simulink model "ex4sima"  (R2018a)
settings: Solver=ode45  StartTime=0.0  StopTime=10  RelTol=1e-3  EnableMultiTasking=on
values from neighbouring files (symbols this model uses):
  A = double(subs(A_sym, symbs, vals))    [load_params.m]
  B = double(subs(B_sym, symbs, vals))    [load_params.m]
  C = double(subs(C_sym, symbs, vals))    [load_params.m]    (also in load_pwm_avg_pred_controller.m = sysd.c; load_pwm_pred_controller.m = sysd.c)
undefined symbols (not defined in the file or in its folder): Ts
settings Model: Creator=BPeixoto  LastModifiedBy=brunolnetto
settings DataIOCC: LimitDataPoints=on  SaveFormat=Array
settings OptimizationCC: LifeSpan=inf
settings DebuggingCC: SFUnexpectedBacktrackingDiag=warning  SFNoUnconditionalDefaultTransitionDiag=warning  SFExecutionAtInitializationDiag=none
settings HardwareCC: ProdBitPerPointer=32  ProdBitPerSizeT=32  ProdBitPerPtrDiffT=32  ProdLargestAtomicFloat=None  ProdIntDivRoundTo=Undefined  ProdEndianess=Unspecified  ProdWordSize=32  ProdHWDeviceType=32-bit Generic
settings ModelReferenceCC: PropagateSignalLabelsOutOfModel=off
settings CodeAppCC: StateflowObjectComments=on
settings GRTTargetCC: TargetLangStandard=C89/C90 (ANSI)  GeneratePreprocessorConditionals=Disable all
settings ConfigComp: CovMetricSettings=dw  CovHtmlReporting=on  CovSaveCumulativeToWorkspaceVar=on  CovSaveSingleToWorkspaceVar=on  CovExternalEMLEnable=off

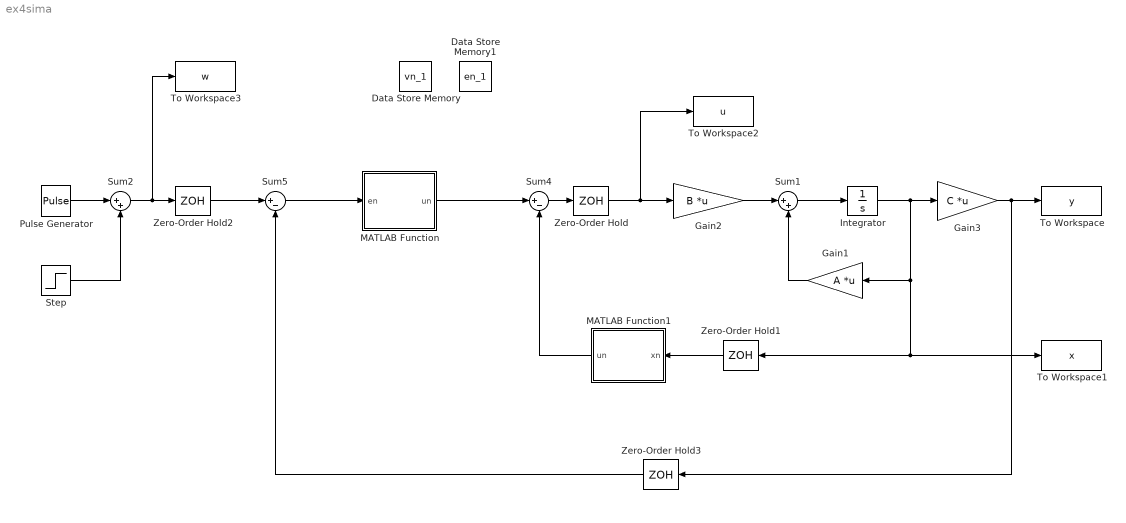
== system ex4sima ==
  Data Store Memory : DataStoreMemory  DataStoreName=vn_1  ShowAdditionalParam=off  OutDataTypeStr=double
  Data Store Memory1 : DataStoreMemory  DataStoreName=en_1  ReadBeforeWriteMsg=warning  WriteAfterWriteMsg=warning  WriteAfterReadMsg=warning  ShowAdditionalParam=off  OutDataTypeStr=double
  Gain1 : Gain  Gain=A  Multiplication=Matrix(K*u) (u vector)
  Gain2 : Gain  Gain=B  Multiplication=Matrix(K*u) (u vector)
  Gain3 : Gain  Gain=C  Multiplication=Matrix(K*u) (u vector)
  Integrator : Integrator  InitialCondition=[0; 0]
  MATLAB Function : MATLAB Function  TreatAsAtomicUnit=on
  MATLAB Function1 : MATLAB Function  TreatAsAtomicUnit=on
  Pulse Generator : DiscretePulseGenerator  PulseType=Time based  Amplitude=0.2  Period=20  PulseWidth=50
  Step : Step  Time=0  After=0.2  SampleTime=0
  Sum1 : Sum  Inputs=|++
  Sum2 : Sum  Inputs=|++
  Sum4 : Sum  Inputs=|+-
  Sum5 : Sum  Inputs=|+-
  To Workspace : ToWorkspace  VariableName=y  SaveFormat=Structure With Time  SampleTime=-1
  To Workspace1 : ToWorkspace  VariableName=x  SaveFormat=Structure With Time  SampleTime=-1
  To Workspace2 : ToWorkspace  VariableName=u  SaveFormat=Structure With Time  SampleTime=-1
  To Workspace3 : ToWorkspace  VariableName=w  SaveFormat=Structure With Time  SampleTime=-1
  Zero-Order Hold : ZeroOrderHold  SampleTime=Ts
  Zero-Order Hold1 : ZeroOrderHold  SampleTime=Ts
  Zero-Order Hold2 : ZeroOrderHold
  Zero-Order Hold3 : ZeroOrderHold  SampleTime=Ts
  wires:
  Sum4/1 -> Zero-Order Hold/1
  Integrator/1 -> Zero-Order Hold1/1, To Workspace1/1, Gain1/1, Gain3/1
  Gain2/1 -> Sum1/1
  Gain3/1 -> Zero-Order Hold3/1, To Workspace/1
  Gain1/1 -> Sum1/2
  Sum1/1 -> Integrator/1
  MATLAB Function/1(un) -> Sum4/1
  Sum5/1 -> MATLAB Function/1(en)
  Zero-Order Hold2/1 -> Sum5/1
  Step/1 -> Sum2/2
  Pulse Generator/1 -> Sum2/1
  Sum2/1 -> Zero-Order Hold2/1, To Workspace3/1
  MATLAB Function1/1(un) -> Sum4/2
  Zero-Order Hold/1 -> To Workspace2/1, Gain2/1
  Zero-Order Hold1/1 -> MATLAB Function1/1(xn)
  Zero-Order Hold3/1 -> Sum5/2

== matlab function ex4sima/MATLAB Function1 ==
  data: xn input; un output; params parameter
function un = integrator(xn, params)
    un = params.K*xn;
end

== matlab function ex4sima/MATLAB Function ==
  data: en input; un output; vn_1 data_store_memory; en_1 data_store_memory; params parameter
function un = integrator(en, params)
    global vn_1;
    global en_1;
    
    vn = vn_1 + en_1;
    
    un = params.Ki*vn;
    
    en_1 = en;
    vn_1 = vn;
end
